simulink model "air_conditioning"  (Simulink 5.0)
settings: Solver=ode45  StartTime=0.0  StopTime=300  RelTol=1e-3
libraries: fuzblock x1
settings Model: LastModifiedBy=Student  BooleanDataType=off

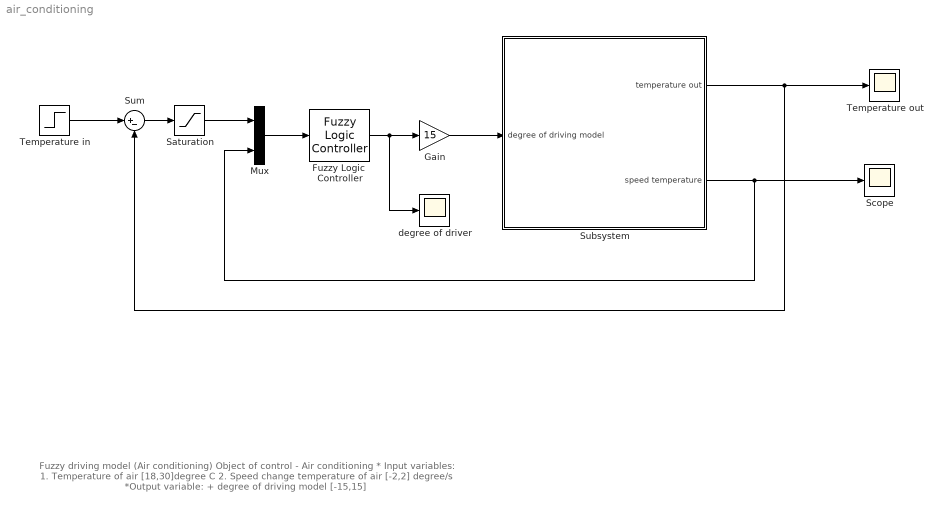
== system air_conditioning ==
  note: Fuzzy driving model (Air conditioning)
      | Object of control - Air conditioning
      | * Input variables:
      |  1. Temperature of air  [18,30]degree C
      |  2. Speed change temperature of air [-2,2] degree/s
      |  *Output variable:
      |  + degree of driving model [-15,15]
  Fuzzy Logic  Controller : fuzblock/Fuzzy Logic  Controller  fis=air_conditioning
  Gain : Gain  Gain=15  SaturateOnIntegerOverflow=on
  Mux : Mux  Inputs=2
  Saturation : Saturate
  Scope : Scope
      settings: TimeRange=300  YMin=-0.8  YMax=1
  Subsystem : Subsystem
  Sum : Sum  Inputs=|+-  SaturateOnIntegerOverflow=on
  Temperature in : Step  After=27  SampleTime=0
  Temperature out : Scope
      settings: TimeRange=250  YMin=15.09  YMax=15.094
  degree of driver : Scope
      settings: TimeRange=250  YMin=15.09  YMax=15.094  SaveName=ScopeData2
  wires:
  Sum/1 -> Saturation/1
  Temperature in/1 -> Sum/1
  Fuzzy Logic  Controller/1 -> Gain/1, degree of driver/1
  Gain/1 -> Subsystem/1(degree of driving model)
  Subsystem/1(temperature out) -> Temperature out/1, Sum/2
  Subsystem/2(speed temperature) -> Scope/1, Mux/2
  Mux/1 -> Fuzzy Logic  Controller/1
  Saturation/1 -> Mux/1

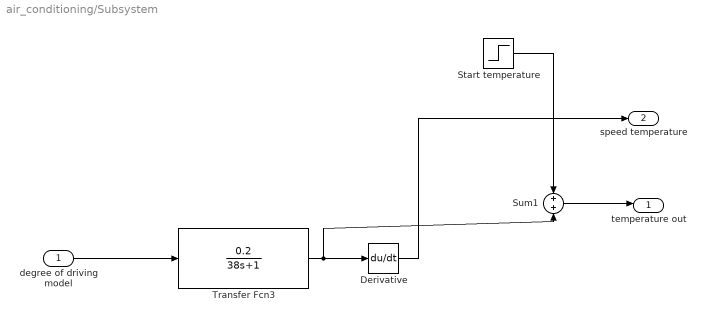
== system air_conditioning/Subsystem ==
  degree of driving model : Inport
  Derivative : Derivative
  Start temperature : Step  Time=0  After=30  SampleTime=0
  Sum1 : Sum  SaturateOnIntegerOverflow=on
  Transfer Fcn3 : TransferFcn  Numerator=[0.2]  Denominator=[38 1]
  temperature out : Outport
  speed temperature : Outport  Port=2
  wires:
  Sum1/1 -> temperature out/1
  degree of driving model/1 -> Transfer Fcn3/1
  Transfer Fcn3/1 -> Derivative/1, Sum1/2
  Derivative/1 -> speed temperature/1
  Start temperature/1 -> Sum1/1
